simulink model "car_speed_control_simulation"  (R2024b)
settings: Solver=VariableStepAuto  StartTime=0.0  StopTime=50  RelTol=1e-3
libraries: simulink_extras x1
settings Model: Creator=USER  LastModifiedBy=USER

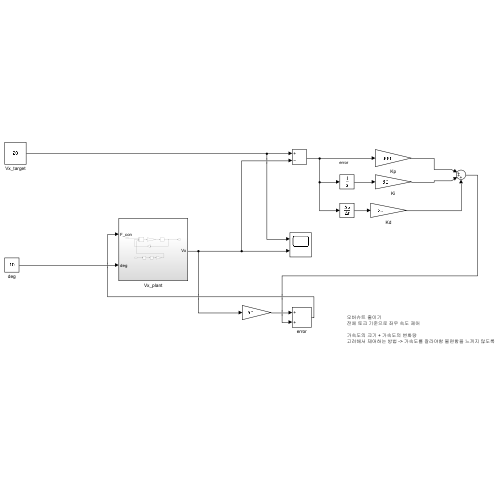
[thumbnail: Simulink's stored preview of the top-level diagram]
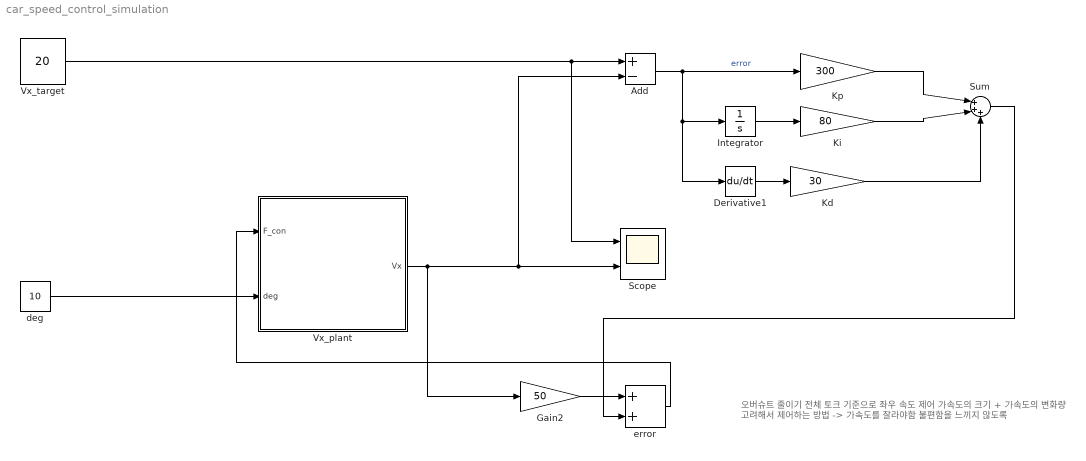
== system car_speed_control_simulation ==
  note: 오버슈트 줄이기
      | 전체 토크 기준으로 좌우 속도 제어
      |
      | 가속도의 크기 + 가속도의 변화량
      | 고려해서 제어하는 방법 -> 가속도를 잘라야함 불편함을 느끼지 않도록
  Add : Sum  Inputs=+-
  Derivative1 : Derivative
  Gain2 : Gain  Gain=50
  Integrator : Integrator
  Kd : Gain  Gain=30
  Ki : Gain  Gain=80
  Kp : Gain  Gain=300
  Scope : Scope  NumInputPorts=2
  Sum : Sum  Inputs=|+++
  Vx_plant : Subsystem
  Vx_target : Constant  Value=20
  deg : Constant  Value=10
  error : Sum
  wires:
  Vx_plant/1(Vx) -> Add/2, Scope/2, Gain2/1
  Vx_target/1 -> Add/1, Scope/1
  Add/1 -> Derivative1/1, Integrator/1, Kp/1  "error"
  Gain2/1 -> error/1
  error/1 -> Vx_plant/1(F_con)
  deg/1 -> Vx_plant/2(deg)
  Integrator/1 -> Ki/1
  Derivative1/1 -> Kd/1
  Kp/1 -> Sum/1
  Ki/1 -> Sum/2
  Kd/1 -> Sum/3
  Sum/1 -> error/2

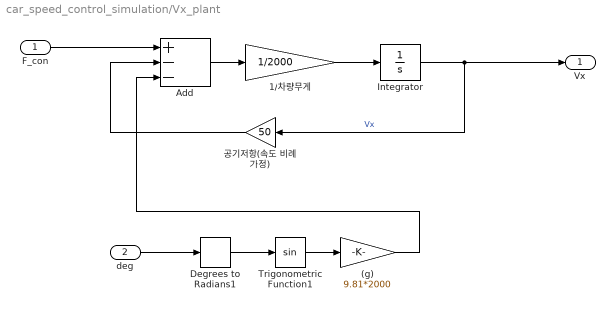
== system car_speed_control_simulation/Vx_plant ==
  F_con : Inport
  deg : Inport  Port=2
  (g) : Gain  Gain=9.81*2000
  1/차량무게 : Gain  Gain=1/2000
  Add : Sum  Inputs=+--
  Degrees to Radians1 : simulink_extras/Transformations/Degrees to Radians
  Integrator : Integrator
  Trigonometric Function1 : Trigonometry
  공기저항(속도 비례 가정) : Gain  Gain=50
  Vx : Outport
  wires:
  Integrator/1 -> Vx/1, 공기저항(속도 비례 가정)/1  "Vx"
  Add/1 -> 1/차량무게/1
  F_con/1 -> Add/1
  1/차량무게/1 -> Integrator/1
  공기저항(속도 비례 가정)/1 -> Add/2
  Degrees to Radians1/1 -> Trigonometric Function1/1
  Trigonometric Function1/1 -> (g)/1
  deg/1 -> Degrees to Radians1/1
  (g)/1 -> Add/3
